simulink model "SolverPlayground"  (R2023a)
settings: Solver=ode15s  StartTime=0.0  StopTime=5  FixedStep=0.001  RelTol=1e-3
settings Model: Creator=Ilya_Andriyanov  LastModifiedBy=ycheb
settings OptimizationCC: ReuseModelBlockBuffer=off

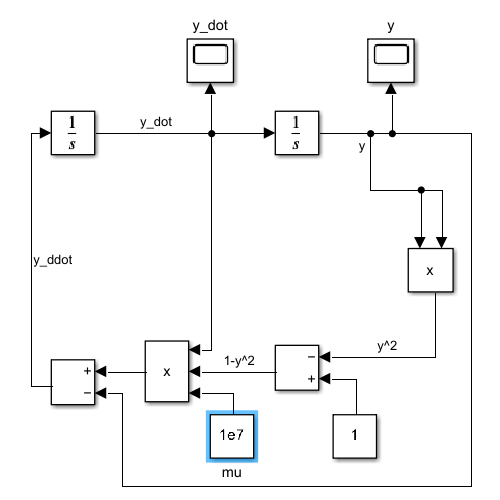
[thumbnail: Simulink's stored preview of the top-level diagram]
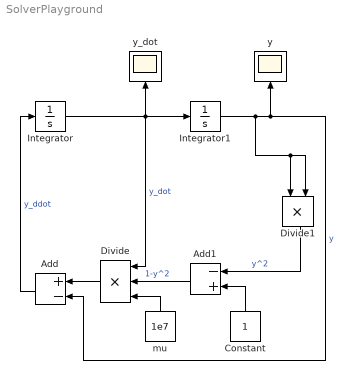
== system SolverPlayground ==
  Add : Sum  Inputs=+-
  Add1 : Sum  Inputs=-+
  Constant : Constant
  Divide : Product  Inputs=***
  Divide1 : Product  Inputs=**
  Integrator : Integrator
  Integrator1 : Integrator  InitialCondition=2
  mu : Constant  Value=1e7
  y : Scope
  y_dot : Scope
  wires:
  Integrator1/1 -> Add/2, y/1, Divide1/2, Divide1/1  "y"
  Divide1/1 -> Add1/1  "y^2"
  Constant/1 -> Add1/2
  mu/1 -> Divide/3
  Add1/1 -> Divide/2  "1-y^2"
  Integrator/1 -> Integrator1/1, y_dot/1, Divide/1  "y_dot"
  Divide/1 -> Add/1
  Add/1 -> Integrator/1  "y_ddot"
